simulink model "modell"  (Simulink 7.3)
settings: Solver=ode4  StartTime=0.0  StopTime=Inf  RelTol=1e-3
values from neighbouring files (symbols this model uses):
  A_w = [zeros(3) eye(3) ... (first row only)    [data.m]
  C_w = [zeros(3) eye(3)]    [data.m]
  D_i = 1*[2    0       0 ... (first row only)    [data.m]
  E_b_i = diag([1 1 1])    [data.m]
  E_b_s = diag([1 1 1])    [data.m]
  K_1 = debug*[diag([-2.2   -2.2    -2.2]) ... (first row only)    [data.m]
  K_2 = debug*0.001*diag([1 1 1])    [data.m]
  K_3 = debug*0.001*diag([0.01 0.01 0.001])    [data.m]
  K_4 = debug*0.001*diag([0.1 0.1 0.1])    [data.m]
  Ke = 100*diag([1.28 1.05 1.28 1.05 2.14])    [data.m]    (also in parameeters.m = diag([1.28 1.05 1.28 1.05 2.14]))
  M_i = 1*[25.8     0       0 ... (first row only)    [data.m]
  pos_0_i = [0, 0, 0]'    [data.m]
  pos_diff = pos_0_s - pos_0_i    [data.m]
  T_i = diag([1000, 1000, 1000])    [data.m]
  T_s = diag([1000, 1000, 1000])    [data.m]
  T_s_inv = T_s^(-1)    [data.m]
  Te = [1     0       1       0       0 ... (first row only)    [data.m]    (also in parameeters.m = [1 0 1 0 0; 0 1 0 1 1; ly1 -lx1 -ly2 -lx2 lx3])
undefined symbols (not defined in the file or in its folder): D, M
libraries: marine_gnc x13, simulink x5, simulink_extras x2
(part 1 of 2)
settings Model: Creator=mcl  LastModifiedBy=mcl  BufferReuse=off
settings OptimizationCC: BlockReduction=off  OptimizeBlockIOStorage=off  BufferReuse=off  ExpressionFolding=off  LocalBlockOutputs=off
settings RTWCC: SystemTargetFile=nidll_vxworks.tlc  TemplateMakefile=nidll_vxworks.tmf  Description=NI Real-Time VxWorks Target for Release 2007b or later  ProcessScript=nidll_vxworks_make_rtw_hook
settings STFCustomTargetCC: MatFileLogging=on  SystemTargetFile=nidll_vxworks.tlc

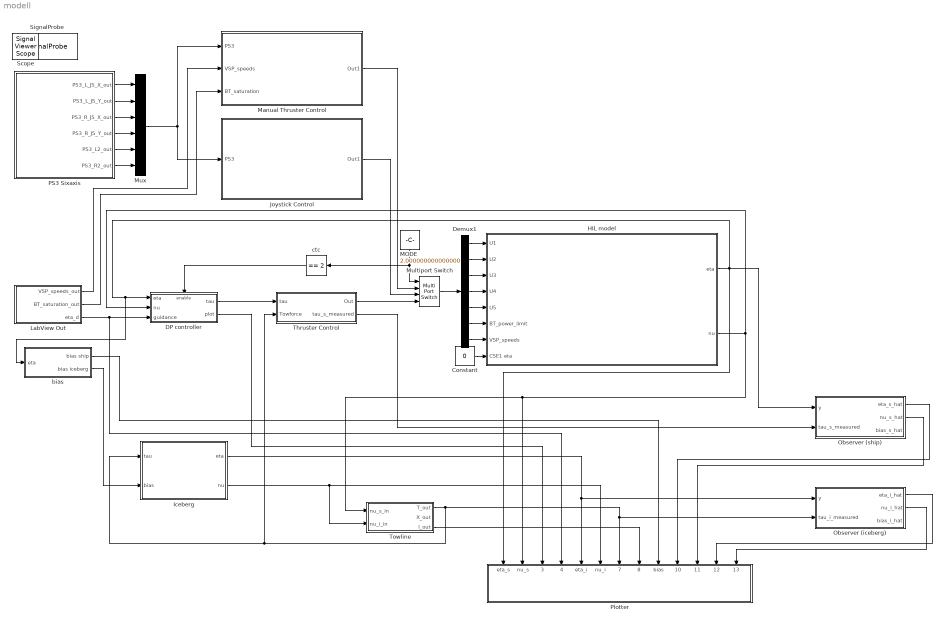
== system modell ==
  Constant : Constant  Value=0  OutDataType=fixdt(1, 16)  OutScaling=2^0
  DP controller : Subsystem
  Demux1 : Demux  Outputs=7
  HIL model : Subsystem
  Iceberg : Subsystem  AncestorBlock=marine_gnc/Examples/Vessels/CyberShipII  LoadFcn=initCS2
      mask Display:
      | image(imread('figs/cs.jpg'))
      | color('white'); port_label('output', 1, 'eta')
      | color('white');port_label('output', 2, 'nu')
      | color('white'); port_label('input', 1, 'tau')
  Joystick Control : Subsystem
  LabView Out : Subsystem
  MODE : Constant  Value=2.000000000000000  OutDataType=fixdt(1, 16)  OutScaling=2^0
  Manual Thruster Control : Subsystem
  Multiport Switch : MultiPortSwitch  zeroidx=on  OutDataType=fixdt(1, 16)  OutScaling=2^0
  Mux : Mux  Inputs=6
  Observer (iceberg) : Subsystem
  Observer (ship) : Subsystem
  PS3 Sixaxis : Subsystem
  Plotter : Subsystem
  SignalProbe : S-Function  Description=Use this block with SIT.  FunctionName=SignalProbe  Parameters=1  EnableBusSupport=off
      settings: PreSaveFcn=NISIT_ModelVars;
      mask Description: The LabVIEW Simulation Interface Toolkit uses the SignalProbe block to probe the signals in the model. The SignalProbe block must be on the top level of the model hierarchy. You can have only one SignalProbe block per model file. Do not rename the SignalProbe block. Do not change the name of another model block to SignalProbe.
  Thruster Control : Subsystem
  Towline : Subsystem
  bias : Subsystem
  ctc : simulink/Logic and Bit Operations/Compare To Constant  SystemSampleTime=-1  relop===  const=2  LogicOutDataTypeMode=uint8
  Scope : SignalViewerScope  IOType=viewer  RefreshTime=0.035000
  wires:
  Demux1/1 -> HIL model/1(U1)
  Demux1/2 -> HIL model/2(U2)
  Demux1/3 -> HIL model/3(U3)
  Demux1/4 -> HIL model/4(U4)
  Demux1/5 -> HIL model/5(U5)
  Demux1/6 -> HIL model/6(BT_power_limit)
  Demux1/7 -> HIL model/7(VSP_speeds)
  Constant/1 -> HIL model/8(CSE1 eta)
  LabView Out/3(eta_d) -> DP controller/3(guidance), Plotter/4(guidance)
  HIL model/1(eta) -> Plotter/1(eta_s), Observer (ship)/1(y), DP controller/1(eta), bias/1(eta)
  HIL model/2(nu) -> Plotter/2(nu_s), Towline/1(nu_s_in), DP controller/2(nu)
  DP controller/1(tau) -> Thruster Control/1(tau)
  DP controller/2(plot) -> Plotter/3(controller)
  Iceberg/1(eta) -> Plotter/5(eta_i), Observer (iceberg)/1(y)
  Iceberg/2(nu) -> Towline/2(nu_i_in), Plotter/6(nu_i)
  Towline/1(T_out) -> Iceberg/1(tau), Thruster Control/2(Towforce), Plotter/7(tow force), Observer (iceberg)/2(tau_i_measured)
  bias/2(bias iceberg) -> Iceberg/2(bias)
  PS3 Sixaxis/1(PS3_L_JS_X_out) -> Mux/1
  PS3 Sixaxis/2(PS3_L_JS_Y_out) -> Mux/2
  PS3 Sixaxis/3(PS3_R_JS_X_out) -> Mux/3
  PS3 Sixaxis/4(PS3_R_JS_Y_out) -> Mux/4
  PS3 Sixaxis/5(PS3_L2_out) -> Mux/5
  PS3 Sixaxis/6(PS3_R2_out) -> Mux/6
  Thruster Control/2(tau_s_measured) -> Observer (ship)/2(tau_s_measured)
  Observer (ship)/1(eta_s_hat) -> Plotter/10(eta_s_hat)
  Observer (ship)/2(nu_s_hat) -> Plotter/11(nu_s_hat)
  Multiport Switch/1 -> Demux1/1
  Thruster Control/1(Out) -> Multiport Switch/4
  MODE/1 -> Multiport Switch/1, ctc/1
  Mux/1 -> Manual Thruster Control/1(PS3), Joystick Control/1(PS3)
  LabView Out/1(VSP_speeds_out) -> Manual Thruster Control/2(VSP_speeds)
  LabView Out/2(BT_saturation_out) -> Manual Thruster Control/3(BT_saturation)
  Manual Thruster Control/1(Out1) -> Multiport Switch/2
  Joystick Control/1(Out1) -> Multiport Switch/3
  ctc/1 -> DP controller/Enable
  Towline/3(l_out) -> Plotter/8(tow length)
  bias/1(bias ship) -> Plotter/9(bias)
  Observer (iceberg)/1(eta_i_hat) -> Plotter/12(eta_i_hat)
  Observer (iceberg)/2(nu_i_hat) -> Plotter/13(nu_i_hat)

== system modell/DP controller ==
  note: eta_d
  eta : Inport  OutDataType=fixdt(1, 16)  OutScaling=2^0
  nu : Inport  Port=2  OutDataType=fixdt(1, 16)  OutScaling=2^0
  guidance : Inport  Port=3  OutDataType=fixdt(1, 16)  OutScaling=2^0
  Enable : EnablePort  StatesWhenEnabling=reset
  DP controller : Subsystem  AncestorBlock="marine_gnc/Control/Dynamic  Positioning /DP controller"  mask(Nonlinear DP Controller){Kp=(0.1)^2*[25.8000 0  0;  0  33.8000  1.0115;  0  1.0115  2.7600 ], Kd=2*0.8*0.1*[25.8000 0  0;  0  33.8000  1.0115;  0  1.0115  2.7600 ], Ki=(0.1^3/10)*[25.8000 0  0;  0  33.8000  1.0115;  0  1.0115  2.7600 ]}
      mask prompts: Kp "Proportional Gain Matrix: Kp"; Kd "Derivative Gain Matrix: Kd"; Ki "Integral Gain Matrix: Ki"
      mask help: Nonlinear PID controller for Set-Point Reulation in Surge, Sway and Yaw
      mask Help:
      | The nonlinear  PID controller uses the rotation matrix in yaw for proper scaling of the surge, sway and yaw gains as a function of the yaw angle.
      | INPUTS: (1) eta_ref, (2) eta, (3) nu. OUPUTS: (1) tau.
      mask Display: disp('Nonlinear PID\n set-point controller')
  tau : Outport  OutDataType=fixdt(1, 16)  OutScaling=2^0
  plot : Outport  Port=2  OutDataType=fixdt(1, 16)  OutScaling=2^0
  wires:
  DP controller/1(tau) -> tau/1, plot/1
  eta/1 -> DP controller/2(eta)
  nu/1 -> DP controller/3(nu)
  guidance/1 -> DP controller/1(eta_ref)

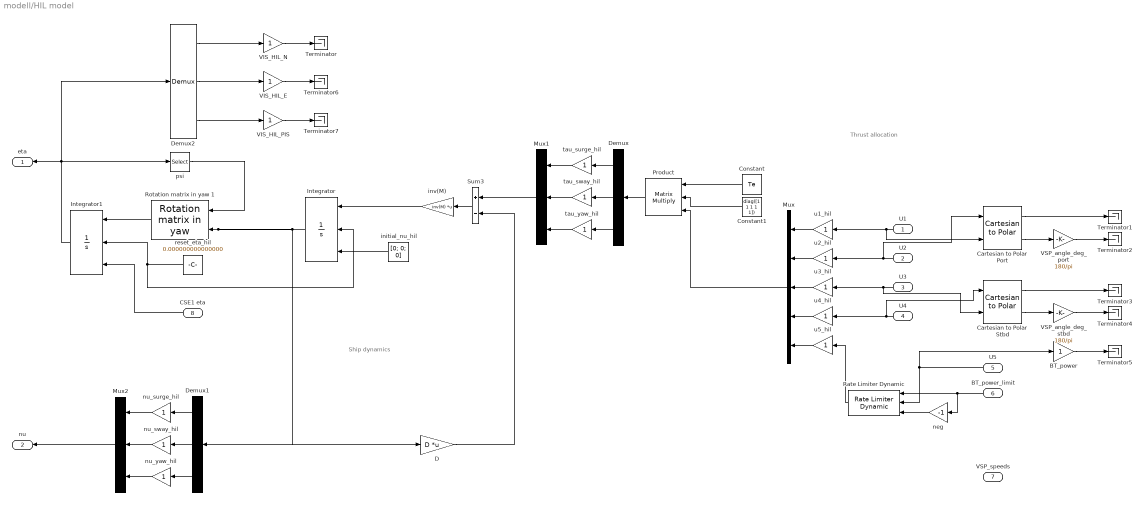
== system modell/HIL model ==
  note: Ship dynamics
  note: Thrust allocation
  U1 : Inport  OutDataType=fixdt(1, 16)  OutScaling=2^0
  U2 : Inport  Port=2  OutDataType=fixdt(1, 16)  OutScaling=2^0
  U3 : Inport  Port=3  OutDataType=fixdt(1, 16)  OutScaling=2^0
  U4 : Inport  Port=4  OutDataType=fixdt(1, 16)  OutScaling=2^0
  U5 : Inport  Port=5  OutDataType=fixdt(1, 16)  OutScaling=2^0
  BT_power_limit : Inport  Port=6  OutDataType=fixdt(1, 16)  OutScaling=2^0
  VSP_speeds : Inport  Port=7  OutDataType=fixdt(1, 16)  OutScaling=2^0
  CSE1 eta : Inport  Port=8  OutDataType=fixdt(1, 16)  OutScaling=2^0
  BT_power : Gain  ParameterDataType=fixdt(1, 16)  ParameterScaling=2^0  OutDataType=fixdt(1, 16)  OutScaling=2^0
  Cartesian to Polar Port : simulink_extras/Transformations/Cartesian to Polar  SystemSampleTime=-1
  Cartesian to Polar Stbd : simulink_extras/Transformations/Cartesian to Polar  SystemSampleTime=-1
  Constant : Constant  Value=Te
  Constant1 : Constant  Value=diag([1 1 1 1 1])
  D : Gain  Gain=D  Multiplication=Matrix(K*u)  ParameterDataType=sfix(16)  ParameterScaling=2^0  OutDataType=sfix(16)  OutScaling=2^0  SaturateOnIntegerOverflow=on  OutDataTypeStr=Inherit: Same as input  ParamDataTypeStr=Inherit: Same as input
  Demux : Demux  Outputs=3
  Demux1 : Demux  Outputs=3
  Demux2 : Demux  Outputs=3
  Integrator : Integrator  ExternalReset=level  InitialConditionSource=external
  Integrator1 : Integrator  ExternalReset=level  InitialConditionSource=external
  Mux : Mux  Inputs=5
  Mux1 : Mux  Inputs=3
  Mux2 : Mux  Inputs=3
  Product : Product  Inputs=3  Multiplication=Matrix(*)  RndMeth=Zero
  Rate Limiter Dynamic : simulink/Discontinuities/Rate Limiter Dynamic  SystemSampleTime=-1
  Rotation matrix in yaw 1 : marine_gnc/Models/ Kinematics/Rotation matrix in yaw   SystemSampleTime=-1
  Sum3 : Sum  Inputs=+-  OutDataType=sfix(16)  OutScaling=2^0  SaturateOnIntegerOverflow=on  InputSameDT=on  OutDataTypeStr=Inherit: Same as first input
  Terminator{,1..7} (8 alike) : Terminator
  VIS_HIL_E : Gain  ParameterDataType=fixdt(1, 16)  ParameterScaling=2^0  OutDataType=fixdt(1, 16)  OutScaling=2^0
  VIS_HIL_N : Gain  ParameterDataType=fixdt(1, 16)  ParameterScaling=2^0  OutDataType=fixdt(1, 16)  OutScaling=2^0
  VIS_HIL_PIS : Gain  ParameterDataType=fixdt(1, 16)  ParameterScaling=2^0  OutDataType=fixdt(1, 16)  OutScaling=2^0
  VSP_angle_deg_port : Gain  Gain=180/pi  ParameterDataType=fixdt(1, 16)  ParameterScaling=2^0  OutDataType=fixdt(1, 16)  OutScaling=2^0
  VSP_angle_deg_stbd : Gain  Gain=180/pi  ParameterDataType=fixdt(1, 16)  ParameterScaling=2^0  OutDataType=fixdt(1, 16)  OutScaling=2^0
  initial_nu_hil : Constant  Value=[0; 0; 0]  OutDataType=fixdt(1, 16)  OutScaling=2^0
  inv(M) : Gain  Gain=inv(M)  Multiplication=Matrix(K*u)  ParameterDataType=sfix(16)  ParameterScaling=2^0  OutDataType=sfix(16)  OutScaling=2^0  SaturateOnIntegerOverflow=on  OutDataTypeStr=Inherit: Same as input  ParamDataTypeStr=Inherit: Same as input
  neg : Gain  Gain=-1  ParameterDataType=fixdt(1, 16)  ParameterScaling=2^0  OutDataType=fixdt(1, 16)  OutScaling=2^0
  nu_surge_hil : Gain  ParameterDataType=fixdt(1, 16)  ParameterScaling=2^0  OutDataType=fixdt(1, 16)  OutScaling=2^0
  nu_sway_hil : Gain  ParameterDataType=fixdt(1, 16)  ParameterScaling=2^0  OutDataType=fixdt(1, 16)  OutScaling=2^0
  nu_yaw_hil : Gain  ParameterDataType=fixdt(1, 16)  ParameterScaling=2^0  OutDataType=fixdt(1, 16)  OutScaling=2^0
  psi : Selector  InputPortWidth=3  IndexOptions=Index vector (dialog)  Indices=[3]  OutputSizes=1
  reset_eta_hil : Constant  Value=0.000000000000000  OutDataType=fixdt(1, 16)  OutScaling=2^0
  tau_surge_hil : Gain  ParameterDataType=fixdt(1, 16)  ParameterScaling=2^0  OutDataType=fixdt(1, 16)  OutScaling=2^0
  tau_sway_hil : Gain  ParameterDataType=fixdt(1, 16)  ParameterScaling=2^0  OutDataType=fixdt(1, 16)  OutScaling=2^0
  tau_yaw_hil : Gain  ParameterDataType=fixdt(1, 16)  ParameterScaling=2^0  OutDataType=fixdt(1, 16)  OutScaling=2^0
  u1_hil : Gain  ParameterDataType=fixdt(1, 16)  ParameterScaling=2^0  OutDataType=fixdt(1, 16)  OutScaling=2^0
  u2_hil : Gain  ParameterDataType=fixdt(1, 16)  ParameterScaling=2^0  OutDataType=fixdt(1, 16)  OutScaling=2^0
  u3_hil : Gain  ParameterDataType=fixdt(1, 16)  ParameterScaling=2^0  OutDataType=fixdt(1, 16)  OutScaling=2^0
  u4_hil : Gain  ParameterDataType=fixdt(1, 16)  ParameterScaling=2^0  OutDataType=fixdt(1, 16)  OutScaling=2^0
  u5_hil : Gain  ParameterDataType=fixdt(1, 16)  ParameterScaling=2^0  OutDataType=fixdt(1, 16)  OutScaling=2^0
  eta : Outport  OutDataType=sfix(16)  OutScaling=2^0
  nu : Outport  Port=2  OutDataType=sfix(16)  OutScaling=2^0
  wires:
  Integrator/1 -> D/1, Demux1/1, Rotation matrix in yaw 1/2
  D/1 -> Sum3/2
  Sum3/1 -> inv(M)/1
  Rotation matrix in yaw 1/1 -> Integrator1/1
  psi/1 -> Rotation matrix in yaw 1/1
  Constant1/1 -> Product/2
  Mux/1 -> Product/3
  Constant/1 -> Product/1
  inv(M)/1 -> Integrator/1
  initial_nu_hil/1 -> Integrator/3
  U1/1 -> u1_hil/1, Cartesian to Polar Port/2
  U2/1 -> u2_hil/1, Cartesian to Polar Port/1
  U3/1 -> u3_hil/1, Cartesian to Polar Stbd/2
  U4/1 -> u4_hil/1, Cartesian to Polar Stbd/1
  Demux/1 -> tau_surge_hil/1
  tau_surge_hil/1 -> Mux1/1
  Demux/2 -> tau_sway_hil/1
  tau_sway_hil/1 -> Mux1/2
  Demux/3 -> tau_yaw_hil/1
  tau_yaw_hil/1 -> Mux1/3
  Product/1 -> Demux/1
  u1_hil/1 -> Mux/1
  u2_hil/1 -> Mux/2
  u3_hil/1 -> Mux/3
  u4_hil/1 -> Mux/4
  u5_hil/1 -> Mux/5
  Demux1/1 -> nu_surge_hil/1
  nu_surge_hil/1 -> Mux2/1
  Demux1/2 -> nu_sway_hil/1
  nu_sway_hil/1 -> Mux2/2
  Demux1/3 -> nu_yaw_hil/1
  nu_yaw_hil/1 -> Mux2/3
  Mux2/1 -> nu/1
  Mux1/1 -> Sum3/1
  Cartesian to Polar Port/1 -> Terminator1/1
  Cartesian to Polar Port/2 -> VSP_angle_deg_port/1
  VSP_angle_deg_port/1 -> Terminator2/1
  Cartesian to Polar Stbd/1 -> Terminator3/1
  Cartesian to Polar Stbd/2 -> VSP_angle_deg_stbd/1
  VSP_angle_deg_stbd/1 -> Terminator4/1
  BT_power/1 -> Terminator5/1
  Integrator1/1 -> psi/1, eta/1, Demux2/1
  reset_eta_hil/1 -> Integrator1/2, Integrator/2
  CSE1 eta/1 -> Integrator1/3
  VIS_HIL_N/1 -> Terminator/1
  Demux2/1 -> VIS_HIL_N/1
  VIS_HIL_E/1 -> Terminator6/1
  VIS_HIL_PIS/1 -> Terminator7/1
  Demux2/2 -> VIS_HIL_E/1
  Demux2/3 -> VIS_HIL_PIS/1
  Rate Limiter Dynamic/1 -> u5_hil/1
  BT_power_limit/1 -> Rate Limiter Dynamic/1, neg/1
  neg/1 -> Rate Limiter Dynamic/3
  U5/1 -> BT_power/1, Rate Limiter Dynamic/2

== system modell/Iceberg ==
  note: nu
  note: nu_dot
  note: etadot
  tau : Inport  OutDataType=sfix(16)  OutScaling=2^0
  bias : Inport  Port=2  OutDataType=fixdt(1, 16)  OutScaling=2^0
  D : Gain  Gain=D_i  Multiplication=Matrix(K*u)  ParameterDataType=sfix(16)  ParameterScaling=2^0  OutDataType=sfix(16)  OutScaling=2^0  SaturateOnIntegerOverflow=on  OutDataTypeStr=Inherit: Same as input  ParamDataTypeStr=Inherit: Same as input
  Integrator1 : Integrator  InitialConditionSource=external
  Integrator2 : Integrator
  Rotation matrix in yaw 1 : marine_gnc/Models/ Kinematics/Rotation matrix in yaw   SystemSampleTime=-1
  Sum3 : Sum  Inputs=+-+  OutDataType=sfix(16)  OutScaling=2^0  SaturateOnIntegerOverflow=on  InputSameDT=on  OutDataTypeStr=Inherit: Same as first input
  initial position : Constant  Value=pos_0_i  OutDataType=fixdt(1, 16)  OutScaling=2^0
  inv(M) : Gain  Gain=inv(M_i)  Multiplication=Matrix(K*u)  ParameterDataType=sfix(16)  ParameterScaling=2^0  OutDataType=sfix(16)  OutScaling=2^0  SaturateOnIntegerOverflow=on  OutDataTypeStr=Inherit: Same as input  ParamDataTypeStr=Inherit: Same as input
  psi : Selector  InputPortWidth=3  IndexOptions=Index vector (dialog)  Indices=[3]  OutputSizes=1
  saturation : Subsystem
  eta : Outport  OutDataType=sfix(16)  OutScaling=2^0
  nu : Outport  Port=2  OutDataType=sfix(16)  OutScaling=2^0
  wires:
  tau/1 -> saturation/1(tau)
  Integrator2/1 -> Rotation matrix in yaw 1/2, nu/1, D/1
  D/1 -> Sum3/2
  Sum3/1 -> inv(M)/1
  inv(M)/1 -> Integrator2/1
  Rotation matrix in yaw 1/1 -> Integrator1/1
  Integrator1/1 -> eta/1, psi/1
  psi/1 -> Rotation matrix in yaw 1/1
  saturation/1(sat_tau) -> Sum3/1
  initial position/1 -> Integrator1/2
  bias/1 -> Sum3/3

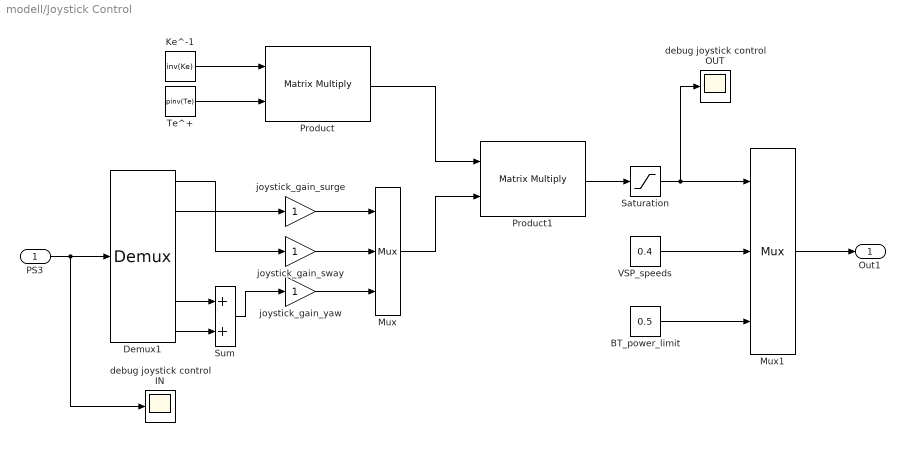
== system modell/Joystick Control ==
  PS3 : Inport  OutDataType=fixdt(1, 16)  OutScaling=2^0
  BT_power_limit : Constant  Value=0.5  OutDataType=fixdt(1, 16)  OutScaling=2^0
  Demux1 : Demux  Outputs=6
  Ke^-1 : Constant  Value=inv(Ke)  OutDataType=fixdt(1, 16)  OutScaling=2^0
  Mux : Mux  Inputs=3
  Mux1 : Mux  Inputs=3
  Product : Product  Multiplication=Matrix(*)  OutDataType=fixdt(1, 16)  OutScaling=2^0  RndMeth=Zero
  Product1 : Product  Multiplication=Matrix(*)  OutDataType=fixdt(1, 16)  OutScaling=2^0  RndMeth=Zero
  Saturation : Saturate  UpperLimit=1.0  LowerLimit=-1.0  OutDataType=fixdt(1, 16)  OutScaling=2^0
  Sum : Sum  OutDataType=fixdt(1, 16)  OutScaling=2^0
  Te^+ : Constant  Value=pinv(Te)  OutDataType=fixdt(1, 16)  OutScaling=2^0
  VSP_speeds : Constant  Value=0.4  OutDataType=fixdt(1, 16)  OutScaling=2^0
  debug joystick control IN : Scope
      settings: YMin=-1.1  YMax=1.1  SaveName=ScopeData17
  debug joystick control OUT : Scope
      settings: YMin=-0.5  YMax=0.65  SaveName=ScopeData16
  joystick_gain_surge : Gain  ParameterDataType=fixdt(1, 16)  ParameterScaling=2^0  OutDataType=fixdt(1, 16)  OutScaling=2^0
  joystick_gain_sway : Gain  ParameterDataType=fixdt(1, 16)  ParameterScaling=2^0  OutDataType=fixdt(1, 16)  OutScaling=2^0
  joystick_gain_yaw : Gain  ParameterDataType=fixdt(1, 16)  ParameterScaling=2^0  OutDataType=fixdt(1, 16)  OutScaling=2^0
  Out1 : Outport  OutDataType=fixdt(1, 16)  OutScaling=2^0
  wires:
  PS3/1 -> Demux1/1, debug joystick control IN/1
  Demux1/1 -> joystick_gain_sway/1
  Demux1/2 -> joystick_gain_surge/1
  Demux1/5 -> Sum/1
  Demux1/6 -> Sum/2
  Sum/1 -> joystick_gain_yaw/1
  Ke^-1/1 -> Product/1
  Te^+/1 -> Product/2
  Product/1 -> Product1/1
  joystick_gain_surge/1 -> Mux/1
  joystick_gain_sway/1 -> Mux/2
  joystick_gain_yaw/1 -> Mux/3
  Mux/1 -> Product1/2
  Mux1/1 -> Out1/1
  VSP_speeds/1 -> Mux1/2
  BT_power_limit/1 -> Mux1/3
  Product1/1 -> Saturation/1
  Saturation/1 -> Mux1/1, debug joystick control OUT/1

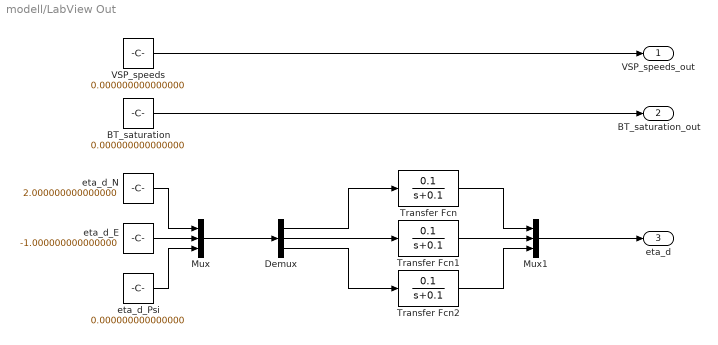
== system modell/LabView Out ==
  BT_saturation : Constant  Value=0.000000000000000  OutDataType=fixdt(1, 16)  OutScaling=2^0
  Demux : Demux  Outputs=3
  Mux : Mux  Inputs=3
  Mux1 : Mux  Inputs=3
  Transfer Fcn : TransferFcn  Numerator=[0.1]  Denominator=[1 0.1]
  Transfer Fcn1 : TransferFcn  Numerator=[0.1]  Denominator=[1 0.1]
  Transfer Fcn2 : TransferFcn  Numerator=[0.1]  Denominator=[1 0.1]
  VSP_speeds : Constant  Value=0.000000000000000  OutDataType=fixdt(1, 16)  OutScaling=2^0
  eta_d_E : Constant  Value=-1.000000000000000  OutDataType=fixdt(1, 16)  OutScaling=2^0
  eta_d_N : Constant  Value=2.000000000000000  OutDataType=fixdt(1, 16)  OutScaling=2^0
  eta_d_Psi : Constant  Value=0.000000000000000  OutDataType=fixdt(1, 16)  OutScaling=2^0
  VSP_speeds_out : Outport  OutDataType=fixdt(1, 16)  OutScaling=2^0
  BT_saturation_out : Outport  Port=2  OutDataType=fixdt(1, 16)  OutScaling=2^0
  eta_d : Outport  Port=3  OutDataType=fixdt(1, 16)  OutScaling=2^0
  wires:
  eta_d_N/1 -> Mux/1
  eta_d_E/1 -> Mux/2
  eta_d_Psi/1 -> Mux/3
  Mux/1 -> Demux/1
  Demux/3 -> Transfer Fcn2/1
  Demux/2 -> Transfer Fcn1/1
  Demux/1 -> Transfer Fcn/1
  Transfer Fcn1/1 -> Mux1/2
  Transfer Fcn2/1 -> Mux1/3
  Transfer Fcn/1 -> Mux1/1
  Mux1/1 -> eta_d/1
  VSP_speeds/1 -> VSP_speeds_out/1
  BT_saturation/1 -> BT_saturation_out/1

== system modell/Manual Thruster Control ==
  PS3 : Inport  OutDataType=fixdt(1, 16)  OutScaling=2^0
  VSP_speeds : Inport  Port=2  OutDataType=fixdt(1, 16)  OutScaling=2^0
  BT_saturation : Inport  Port=3  OutDataType=fixdt(1, 16)  OutScaling=2^0
  Demux1 : Demux  Outputs=6
  Mux : Mux  Inputs=7
  Sum : Sum  OutDataType=fixdt(1, 16)  OutScaling=2^0
  U{1..5} (5 alike) : Gain  ParameterDataType=fixdt(1, 16)  ParameterScaling=2^0  OutDataType=fixdt(1, 16)  OutScaling=2^0
  Out1 : Outport  OutDataType=fixdt(1, 16)  OutScaling=2^0
  wires:
  Mux/1 -> Out1/1
  PS3/1 -> Demux1/1
  Demux1/5 -> Sum/1
  Demux1/6 -> Sum/2
  Sum/1 -> U5/1
  BT_saturation/1 -> Mux/6
  VSP_speeds/1 -> Mux/7
  U1/1 -> Mux/1
  U2/1 -> Mux/2
  U3/1 -> Mux/3
  U4/1 -> Mux/4
  U5/1 -> Mux/5
  Demux1/2 -> U1/1
  Demux1/1 -> U2/1
  Demux1/4 -> U3/1
  Demux1/3 -> U4/1

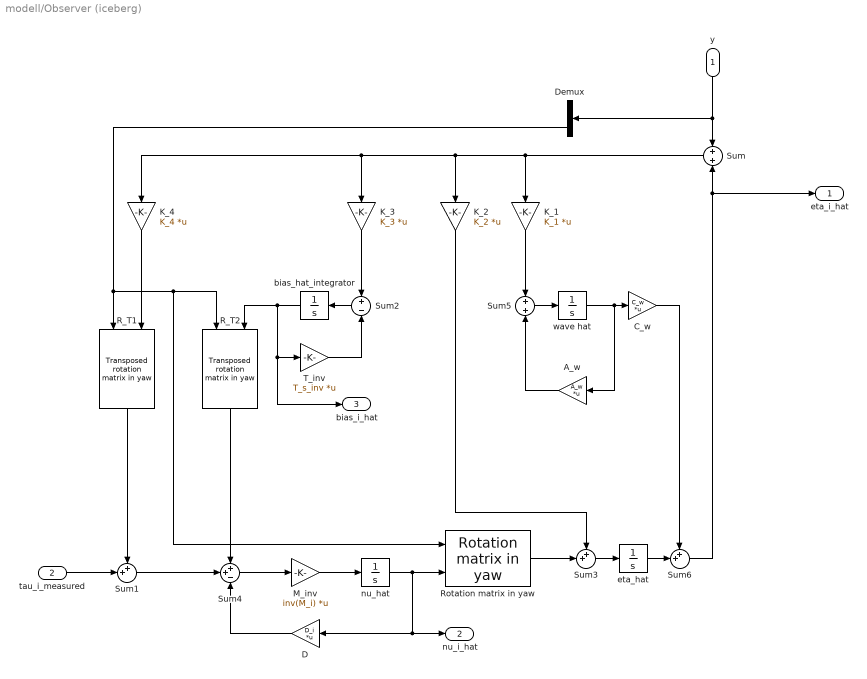
== system modell/Observer (iceberg) ==
  y : Inport  OutDataType=fixdt(1, 16)  OutScaling=2^0
  tau_i_measured : Inport  Port=2  OutDataType=fixdt(1, 16)  OutScaling=2^0
  A_w : Gain  Gain=A_w  Multiplication=Matrix(K*u)  ParameterDataType=fixdt(1, 16)  ParameterScaling=2^0  OutDataType=fixdt(1, 16)  OutScaling=2^0
  C_w : Gain  Gain=C_w  Multiplication=Matrix(K*u)  ParameterDataType=fixdt(1, 16)  ParameterScaling=2^0  OutDataType=fixdt(1, 16)  OutScaling=2^0
  D : Gain  Gain=D_i  Multiplication=Matrix(K*u)  ParameterDataType=fixdt(1, 16)  ParameterScaling=2^0  OutDataType=fixdt(1, 16)  OutScaling=2^0
  Demux : Demux  Outputs=3
  K_1 : Gain  Gain=K_1  Multiplication=Matrix(K*u)  ParameterDataType=fixdt(1, 16)  ParameterScaling=2^0  OutDataType=fixdt(1, 16)  OutScaling=2^0
  K_2 : Gain  Gain=K_2  Multiplication=Matrix(K*u)  ParameterDataType=fixdt(1, 16)  ParameterScaling=2^0  OutDataType=fixdt(1, 16)  OutScaling=2^0
  K_3 : Gain  Gain=K_3  Multiplication=Matrix(K*u)  ParameterDataType=fixdt(1, 16)  ParameterScaling=2^0  OutDataType=fixdt(1, 16)  OutScaling=2^0
  K_4 : Gain  Gain=K_4  Multiplication=Matrix(K*u)  ParameterDataType=fixdt(1, 16)  ParameterScaling=2^0  OutDataType=fixdt(1, 16)  OutScaling=2^0
  M_inv : Gain  Gain=inv(M_i)  Multiplication=Matrix(K*u)  ParameterDataType=fixdt(1, 16)  ParameterScaling=2^0  OutDataType=fixdt(1, 16)  OutScaling=2^0
  R_T1 : marine_gnc/Models/ Kinematics/Transposed rotation  matrix in yaw  SystemSampleTime=-1
  R_T2 : marine_gnc/Models/ Kinematics/Transposed rotation  matrix in yaw  SystemSampleTime=-1
  "Rotation matrix in yaw " : marine_gnc/Models/ Kinematics/Rotation matrix in yaw   SystemSampleTime=-1
  Sum : Sum  OutDataType=fixdt(1, 16)  OutScaling=2^0
  Sum1 : Sum  Inputs=++|  OutDataType=fixdt(1, 16)  OutScaling=2^0
  Sum2 : Sum  Inputs=+-  OutDataType=fixdt(1, 16)  OutScaling=2^0
  Sum3 : Sum  Inputs=++|  OutDataType=fixdt(1, 16)  OutScaling=2^0
  Sum4 : Sum  Inputs=++-  OutDataType=fixdt(1, 16)  OutScaling=2^0
  Sum5 : Sum  OutDataType=fixdt(1, 16)  OutScaling=2^0
  Sum6 : Sum  Inputs=++|  OutDataType=fixdt(1, 16)  OutScaling=2^0
  T_inv : Gain  Gain=T_s_inv  Multiplication=Matrix(K*u)  ParameterDataType=fixdt(1, 16)  ParameterScaling=2^0  OutDataType=fixdt(1, 16)  OutScaling=2^0
  bias_hat_integrator : Integrator
  eta_hat : Integrator
  nu_hat : Integrator
  wave hat : Integrator
  eta_i_hat : Outport  OutDataType=fixdt(1, 16)  OutScaling=2^0
  nu_i_hat : Outport  Port=2  OutDataType=fixdt(1, 16)  OutScaling=2^0
  bias_i_hat : Outport  Port=3  OutDataType=fixdt(1, 16)  OutScaling=2^0
  wires:
  tau_i_measured/1 -> Sum1/2
  y/1 -> Sum/1, Demux/1
  Sum/1 -> K_4/1, K_3/1, K_2/1, K_1/1
  K_4/1 -> R_T1/2
  R_T1/1 -> Sum1/1
  Demux/3 -> R_T1/1, R_T2/1, "Rotation matrix in yaw "/1
  R_T2/1 -> Sum4/1
  Sum1/1 -> Sum4/2
  K_3/1 -> Sum2/1
  T_inv/1 -> Sum2/2
  Sum2/1 -> bias_hat_integrator/1
  bias_hat_integrator/1 -> R_T2/2, T_inv/1, bias_i_hat/1
  Sum4/1 -> M_inv/1
  M_inv/1 -> nu_hat/1
  nu_hat/1 -> "Rotation matrix in yaw "/2, D/1, nu_i_hat/1
  D/1 -> Sum4/3
  "Rotation matrix in yaw "/1 -> Sum3/2
  K_2/1 -> Sum3/1
  K_1/1 -> Sum5/1
  Sum5/1 -> wave hat/1
  A_w/1 -> Sum5/2
  wave hat/1 -> C_w/1, A_w/1
  Sum3/1 -> eta_hat/1
  eta_hat/1 -> Sum6/2
  Sum6/1 -> Sum/2, eta_i_hat/1
  C_w/1 -> Sum6/1

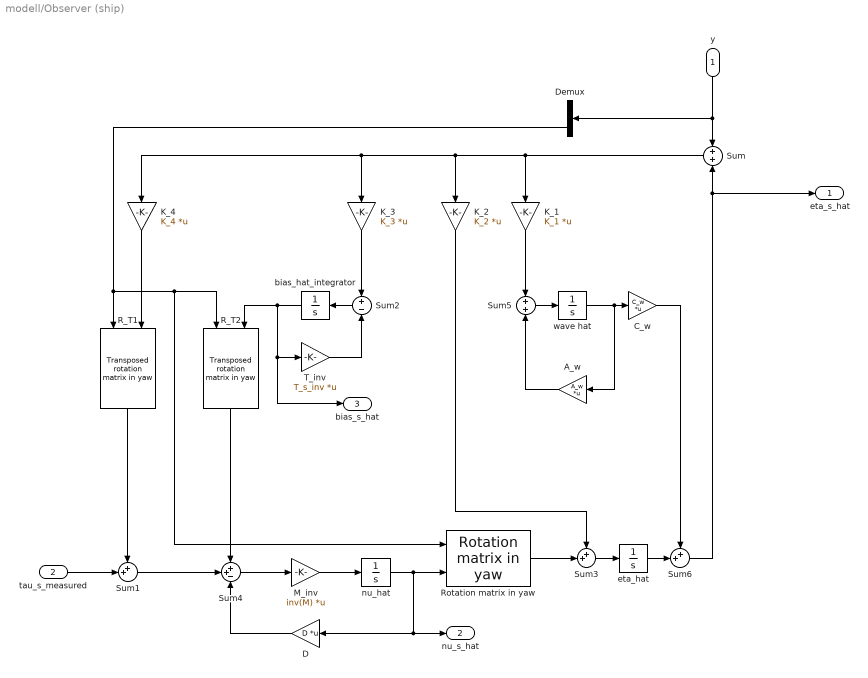
== system modell/Observer (ship) ==
  y : Inport  OutDataType=fixdt(1, 16)  OutScaling=2^0
  tau_s_measured : Inport  Port=2  OutDataType=fixdt(1, 16)  OutScaling=2^0
  A_w : Gain  Gain=A_w  Multiplication=Matrix(K*u)  ParameterDataType=fixdt(1, 16)  ParameterScaling=2^0  OutDataType=fixdt(1, 16)  OutScaling=2^0
  C_w : Gain  Gain=C_w  Multiplication=Matrix(K*u)  ParameterDataType=fixdt(1, 16)  ParameterScaling=2^0  OutDataType=fixdt(1, 16)  OutScaling=2^0
  D : Gain  Gain=D  Multiplication=Matrix(K*u)  ParameterDataType=fixdt(1, 16)  ParameterScaling=2^0  OutDataType=fixdt(1, 16)  OutScaling=2^0
  Demux : Demux  Outputs=3
  K_1 : Gain  Gain=K_1  Multiplication=Matrix(K*u)  ParameterDataType=fixdt(1, 16)  ParameterScaling=2^0  OutDataType=fixdt(1, 16)  OutScaling=2^0
  K_2 : Gain  Gain=K_2  Multiplication=Matrix(K*u)  ParameterDataType=fixdt(1, 16)  ParameterScaling=2^0  OutDataType=fixdt(1, 16)  OutScaling=2^0
  K_3 : Gain  Gain=K_3  Multiplication=Matrix(K*u)  ParameterDataType=fixdt(1, 16)  ParameterScaling=2^0  OutDataType=fixdt(1, 16)  OutScaling=2^0
  K_4 : Gain  Gain=K_4  Multiplication=Matrix(K*u)  ParameterDataType=fixdt(1, 16)  ParameterScaling=2^0  OutDataType=fixdt(1, 16)  OutScaling=2^0
  M_inv : Gain  Gain=inv(M)  Multiplication=Matrix(K*u)  ParameterDataType=fixdt(1, 16)  ParameterScaling=2^0  OutDataType=fixdt(1, 16)  OutScaling=2^0
  R_T1 : marine_gnc/Models/ Kinematics/Transposed rotation  matrix in yaw  SystemSampleTime=-1
  R_T2 : marine_gnc/Models/ Kinematics/Transposed rotation  matrix in yaw  SystemSampleTime=-1
  "Rotation matrix in yaw " : marine_gnc/Models/ Kinematics/Rotation matrix in yaw   SystemSampleTime=-1
  Sum : Sum  OutDataType=fixdt(1, 16)  OutScaling=2^0
  Sum1 : Sum  Inputs=++|  OutDataType=fixdt(1, 16)  OutScaling=2^0
  Sum2 : Sum  Inputs=+-  OutDataType=fixdt(1, 16)  OutScaling=2^0
  Sum3 : Sum  Inputs=++|  OutDataType=fixdt(1, 16)  OutScaling=2^0
  Sum4 : Sum  Inputs=++-  OutDataType=fixdt(1, 16)  OutScaling=2^0
  Sum5 : Sum  OutDataType=fixdt(1, 16)  OutScaling=2^0
  Sum6 : Sum  Inputs=++|  OutDataType=fixdt(1, 16)  OutScaling=2^0
  T_inv : Gain  Gain=T_s_inv  Multiplication=Matrix(K*u)  ParameterDataType=fixdt(1, 16)  ParameterScaling=2^0  OutDataType=fixdt(1, 16)  OutScaling=2^0
  bias_hat_integrator : Integrator
  eta_hat : Integrator
  nu_hat : Integrator
  wave hat : Integrator
  eta_s_hat : Outport  OutDataType=fixdt(1, 16)  OutScaling=2^0
  nu_s_hat : Outport  Port=2  OutDataType=fixdt(1, 16)  OutScaling=2^0
  bias_s_hat : Outport  Port=3  OutDataType=fixdt(1, 16)  OutScaling=2^0
  wires:
  tau_s_measured/1 -> Sum1/2
  y/1 -> Sum/1, Demux/1
  Sum/1 -> K_4/1, K_3/1, K_2/1, K_1/1
  K_4/1 -> R_T1/2
  R_T1/1 -> Sum1/1
  Demux/3 -> R_T1/1, R_T2/1, "Rotation matrix in yaw "/1
  R_T2/1 -> Sum4/1
  Sum1/1 -> Sum4/2
  K_3/1 -> Sum2/1
  T_inv/1 -> Sum2/2
  Sum2/1 -> bias_hat_integrator/1
  bias_hat_integrator/1 -> R_T2/2, T_inv/1, bias_s_hat/1
  Sum4/1 -> M_inv/1
  M_inv/1 -> nu_hat/1
  nu_hat/1 -> "Rotation matrix in yaw "/2, D/1, nu_s_hat/1
  D/1 -> Sum4/3
  "Rotation matrix in yaw "/1 -> Sum3/2
  K_2/1 -> Sum3/1
  K_1/1 -> Sum5/1
  Sum5/1 -> wave hat/1
  A_w/1 -> Sum5/2
  wave hat/1 -> C_w/1, A_w/1
  Sum3/1 -> eta_hat/1
  eta_hat/1 -> Sum6/2
  Sum6/1 -> Sum/2, eta_s_hat/1
  C_w/1 -> Sum6/1

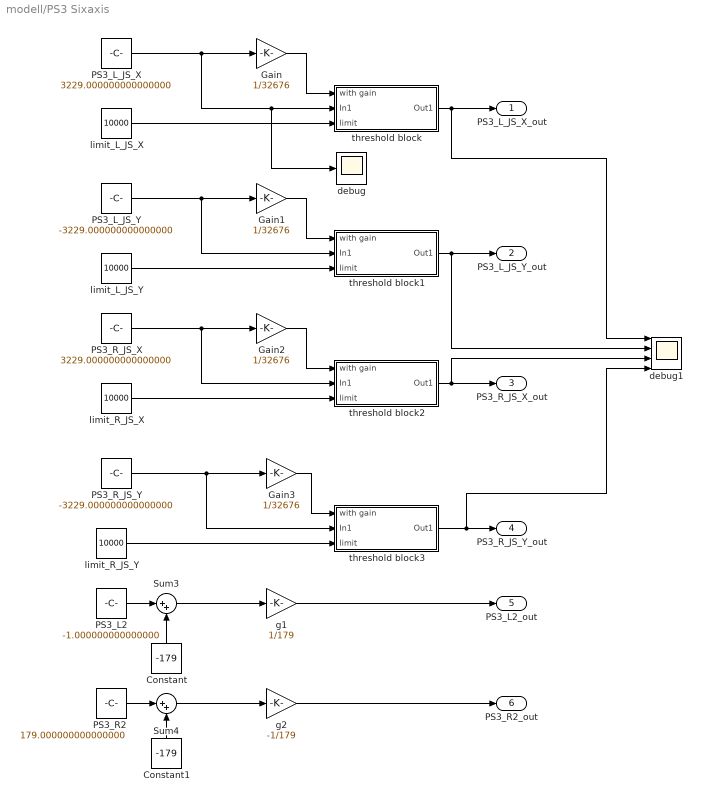
== system modell/PS3 Sixaxis ==
  Constant : Constant  Value=-179  OutDataType=fixdt(1, 16)  OutScaling=2^0
  Constant1 : Constant  Value=-179  OutDataType=fixdt(1, 16)  OutScaling=2^0
  Gain{,1..3} (4 alike) : Gain  Gain=1/32676  ParameterDataType=fixdt(1, 16)  ParameterScaling=2^0  OutDataType=fixdt(1, 16)  OutScaling=2^0
  PS3_L2 : Constant  Value=-1.000000000000000  OutDataType=fixdt(1, 16)  OutScaling=2^0
  PS3_L_JS_X : Constant  Value=3229.000000000000000  OutDataType=fixdt(1, 16)  OutScaling=2^0
  PS3_L_JS_Y : Constant  Value=-3229.000000000000000  OutDataType=fixdt(1, 16)  OutScaling=2^0
  PS3_R2 : Constant  Value=179.000000000000000  OutDataType=fixdt(1, 16)  OutScaling=2^0
  PS3_R_JS_X : Constant  Value=3229.000000000000000  OutDataType=fixdt(1, 16)  OutScaling=2^0
  PS3_R_JS_Y : Constant  Value=-3229.000000000000000  OutDataType=fixdt(1, 16)  OutScaling=2^0
  Sum3 : Sum  Inputs=|++  OutDataType=fixdt(1, 16)  OutScaling=2^0
  Sum4 : Sum  Inputs=|++  OutDataType=fixdt(1, 16)  OutScaling=2^0
  debug : Scope
      settings: YMin=3513  YMax=3513  SaveName=ScopeData9
  debug1 : Scope  NumInputPorts=4
      settings: YMin=-1~-1~-1~-1  YMax=1~1~1~1  SaveName=ScopeData10
  g1 : Gain  Gain=1/179  ParameterDataType=fixdt(1, 16)  ParameterScaling=2^0  OutDataType=fixdt(1, 16)  OutScaling=2^0
  g2 : Gain  Gain=-1/179  ParameterDataType=fixdt(1, 16)  ParameterScaling=2^0  OutDataType=fixdt(1, 16)  OutScaling=2^0
  limit_L_JS_X : Constant  Value=10000  OutDataType=fixdt(1, 16)  OutScaling=2^0
  limit_L_JS_Y : Constant  Value=10000  OutDataType=fixdt(1, 16)  OutScaling=2^0
  limit_R_JS_X : Constant  Value=10000  OutDataType=fixdt(1, 16)  OutScaling=2^0
  limit_R_JS_Y : Constant  Value=10000  OutDataType=fixdt(1, 16)  OutScaling=2^0
  threshold block : Subsystem
  threshold block1 : Subsystem
  threshold block2 : Subsystem
  threshold block3 : Subsystem
  PS3_L_JS_X_out : Outport  OutDataType=fixdt(1, 16)  OutScaling=2^0
  PS3_L_JS_Y_out : Outport  Port=2  OutDataType=fixdt(1, 16)  OutScaling=2^0
  PS3_R_JS_X_out : Outport  Port=3  OutDataType=fixdt(1, 16)  OutScaling=2^0
  PS3_R_JS_Y_out : Outport  Port=4  OutDataType=fixdt(1, 16)  OutScaling=2^0
  PS3_L2_out : Outport  Port=5  OutDataType=fixdt(1, 16)  OutScaling=2^0
  PS3_R2_out : Outport  Port=6  OutDataType=fixdt(1, 16)  OutScaling=2^0
  wires:
  PS3_L_JS_Y/1 -> Gain1/1, threshold block1/2(In1)
  PS3_L_JS_X/1 -> Gain/1, threshold block/2(In1), debug/1
  PS3_R_JS_Y/1 -> Gain3/1, threshold block3/2(In1)
  PS3_R_JS_X/1 -> Gain2/1, threshold block2/2(In1)
  PS3_L2/1 -> Sum3/1
  Sum3/1 -> g1/1
  PS3_R2/1 -> Sum4/1
  Sum4/1 -> g2/1
  threshold block/1(Out1) -> debug1/1, PS3_L_JS_X_out/1
  Gain/1 -> threshold block/1(with gain)
  Gain1/1 -> threshold block1/1(with gain)
  threshold block1/1(Out1) -> debug1/2, PS3_L_JS_Y_out/1
  Gain2/1 -> threshold block2/1(with gain)
  threshold block2/1(Out1) -> debug1/3, PS3_R_JS_X_out/1
  Gain3/1 -> threshold block3/1(with gain)
  threshold block3/1(Out1) -> debug1/4, PS3_R_JS_Y_out/1
  limit_L_JS_X/1 -> threshold block/3(limit)
  limit_L_JS_Y/1 -> threshold block1/3(limit)
  limit_R_JS_X/1 -> threshold block2/3(limit)
  limit_R_JS_Y/1 -> threshold block3/3(limit)
  g1/1 -> PS3_L2_out/1
  g2/1 -> PS3_R2_out/1
  Constant/1 -> Sum3/2
  Constant1/1 -> Sum4/2

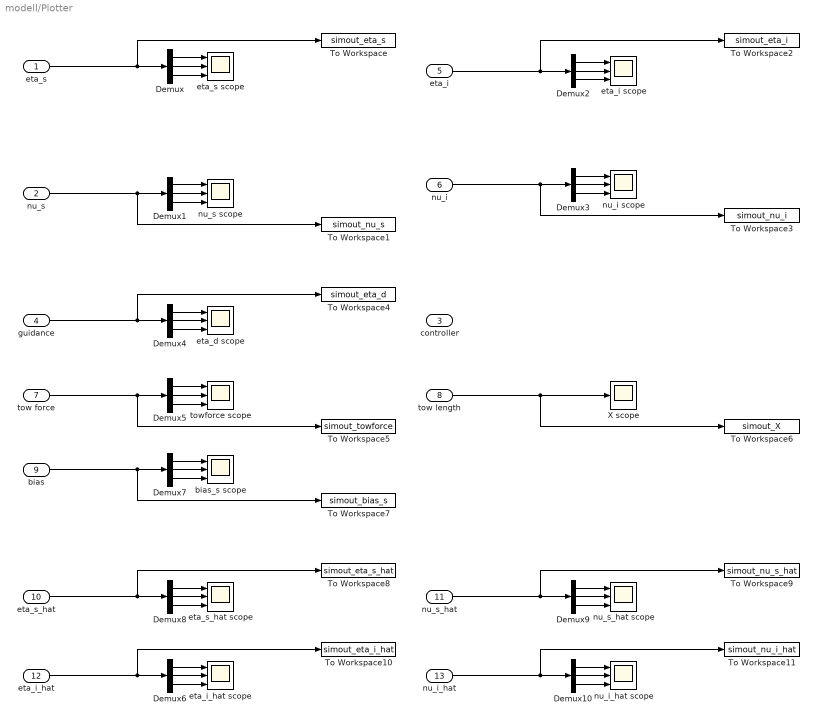
== system modell/Plotter ==
  eta_s : Inport  OutDataType=fixdt(1, 16)  OutScaling=2^0
  nu_s : Inport  Port=2  OutDataType=fixdt(1, 16)  OutScaling=2^0
  controller : Inport  Port=3  OutDataType=fixdt(1, 16)  OutScaling=2^0
  guidance : Inport  Port=4  OutDataType=fixdt(1, 16)  OutScaling=2^0
  eta_i : Inport  Port=5  OutDataType=fixdt(1, 16)  OutScaling=2^0
  nu_i : Inport  Port=6  OutDataType=fixdt(1, 16)  OutScaling=2^0
  tow force : Inport  Port=7  OutDataType=fixdt(1, 16)  OutScaling=2^0
  tow length : Inport  Port=8  OutDataType=fixdt(1, 16)  OutScaling=2^0
  bias : Inport  Port=9  OutDataType=fixdt(1, 16)  OutScaling=2^0
  eta_s_hat : Inport  Port=10  OutDataType=fixdt(1, 16)  OutScaling=2^0
  nu_s_hat : Inport  Port=11  OutDataType=fixdt(1, 16)  OutScaling=2^0
  eta_i_hat : Inport  Port=12  OutDataType=fixdt(1, 16)  OutScaling=2^0
  nu_i_hat : Inport  Port=13  OutDataType=fixdt(1, 16)  OutScaling=2^0
  Demux{,1..10} (11 alike) : Demux  Outputs=3
  To Workspace : ToWorkspace  VariableName=simout_eta_s  SampleTime=-1  SaveFormat=Structure With Time
  To Workspace1 : ToWorkspace  VariableName=simout_nu_s  SampleTime=-1  SaveFormat=Structure
  To Workspace10 : ToWorkspace  VariableName=simout_eta_i_hat  SampleTime=-1  SaveFormat=Structure
  To Workspace11 : ToWorkspace  VariableName=simout_nu_i_hat  SampleTime=-1  SaveFormat=Structure
  To Workspace2 : ToWorkspace  VariableName=simout_eta_i  SampleTime=-1  SaveFormat=Structure
  To Workspace3 : ToWorkspace  VariableName=simout_nu_i  SampleTime=-1  SaveFormat=Structure
  To Workspace4 : ToWorkspace  VariableName=simout_eta_d  SampleTime=-1  SaveFormat=Structure
  To Workspace5 : ToWorkspace  VariableName=simout_towforce  SampleTime=-1  SaveFormat=Structure
  To Workspace6 : ToWorkspace  VariableName=simout_X  SampleTime=-1  SaveFormat=Structure
  To Workspace7 : ToWorkspace  VariableName=simout_bias_s  SampleTime=-1  SaveFormat=Structure
  To Workspace8 : ToWorkspace  VariableName=simout_eta_s_hat  SampleTime=-1  SaveFormat=Structure
  To Workspace9 : ToWorkspace  VariableName=simout_nu_s_hat  SampleTime=-1  SaveFormat=Structure
  X scope : Scope
      settings: YMin=10  YMax=30  SaveName=ScopeData6
  bias_s scope : Scope  NumInputPorts=3
      settings: YMin=-2.5~-2.5~-2.5  YMax=0.75~0.75~0.75  SaveName=ScopeData8
  eta_d scope : Scope  NumInputPorts=3
      settings: YMin=-5~-5~-5  YMax=5~5~5  SaveName=ScopeData4
  eta_i scope : Scope  NumInputPorts=3
      settings: YMin=-5~-5~-5  YMax=5~5~5  SaveName=ScopeData2
  eta_i_hat scope : Scope  NumInputPorts=3
      settings: YMin=8.55~-0.0015~-0.00225  YMax=9.45~0.001~0.0025  SaveName=ScopeData14
  eta_s scope : Scope  NumInputPorts=3
      settings: YMin=8.55~-0.0015~-0.00225  YMax=9.45~0.001~0.0025
  eta_s_hat scope : Scope  NumInputPorts=3
      settings: YMin=8.55~-0.0015~-0.00225  YMax=9.45~0.001~0.0025  SaveName=ScopeData11
  nu_i scope : Scope  NumInputPorts=3
      settings: YMin=-5~-5~-5  YMax=5~5~5  SaveName=ScopeData3
  nu_i_hat scope : Scope  NumInputPorts=3
      settings: YMin=8.55~-0.0015~-0.00225  YMax=9.45~0.001~0.0025  SaveName=ScopeData15
  nu_s scope : Scope  NumInputPorts=3
      settings: YMin=-5~-5~-5  YMax=5~5~5
  nu_s_hat scope : Scope  NumInputPorts=3
      settings: YMin=8.55~-0.0015~-0.00225  YMax=9.45~0.001~0.0025  SaveName=ScopeData12
  towforce scope : Scope  NumInputPorts=3
      settings: YMin=9~-3.51e-021~-1  YMax=27~-3.47e-021~1  SaveName=ScopeData5
  wires:
  eta_s/1 -> Demux/1, To Workspace/1
  Demux/1 -> eta_s scope/1
  Demux/2 -> eta_s scope/2
  Demux/3 -> eta_s scope/3
  nu_s/1 -> Demux1/1, To Workspace1/1
  Demux1/1 -> nu_s scope/1
  Demux1/2 -> nu_s scope/2
  Demux1/3 -> nu_s scope/3
  eta_i/1 -> Demux2/1, To Workspace2/1
  Demux2/1 -> eta_i scope/1
  Demux2/2 -> eta_i scope/2
  Demux2/3 -> eta_i scope/3
  nu_i/1 -> Demux3/1, To Workspace3/1
  Demux3/1 -> nu_i scope/1
  Demux3/2 -> nu_i scope/2
  Demux3/3 -> nu_i scope/3
  guidance/1 -> Demux4/1, To Workspace4/1
  Demux4/1 -> eta_d scope/1
  Demux4/2 -> eta_d scope/2
  Demux4/3 -> eta_d scope/3
  tow force/1 -> Demux5/1, To Workspace5/1
  Demux5/1 -> towforce scope/1
  Demux5/2 -> towforce scope/2
  Demux5/3 -> towforce scope/3
  tow length/1 -> To Workspace6/1, X scope/1
  bias/1 -> Demux7/1, To Workspace7/1
  Demux7/1 -> bias_s scope/1
  Demux7/2 -> bias_s scope/2
  Demux7/3 -> bias_s scope/3
  eta_s_hat/1 -> Demux8/1, To Workspace8/1
  Demux8/1 -> eta_s_hat scope/1
  Demux8/2 -> eta_s_hat scope/2
  Demux8/3 -> eta_s_hat scope/3
  nu_s_hat/1 -> Demux9/1, To Workspace9/1
  Demux9/1 -> nu_s_hat scope/1
  Demux9/2 -> nu_s_hat scope/2
  Demux9/3 -> nu_s_hat scope/3
  eta_i_hat/1 -> Demux6/1, To Workspace10/1
  Demux6/1 -> eta_i_hat scope/1
  Demux6/2 -> eta_i_hat scope/2
  Demux6/3 -> eta_i_hat scope/3
  nu_i_hat/1 -> Demux10/1, To Workspace11/1
  Demux10/1 -> nu_i_hat scope/1
  Demux10/2 -> nu_i_hat scope/2
  Demux10/3 -> nu_i_hat scope/3

== system modell/Thruster Control ==
  tau : Inport  OutDataType=fixdt(1, 16)  OutScaling=2^0
  Towforce : Inport  Port=2  OutDataType=fixdt(1, 16)  OutScaling=2^0
  BT_power_limit : Constant  Value=0.5  OutDataType=fixdt(1, 16)  OutScaling=2^0
  Ke^-1 : Constant  Value=inv(Ke)  OutDataType=fixdt(1, 16)  OutScaling=2^0
  Mux1 : Mux  Inputs=3
  Product : Product  Multiplication=Matrix(*)  OutDataType=fixdt(1, 16)  OutScaling=2^0  RndMeth=Zero
  Product1 : Product  Multiplication=Matrix(*)  OutDataType=fixdt(1, 16)  OutScaling=2^0  RndMeth=Zero
  Saturation : Saturate  UpperLimit=1.0  LowerLimit=-1.0  OutDataType=fixdt(1, 16)  OutScaling=2^0
  Sum : Sum  Inputs=|+-  OutDataType=fixdt(1, 16)  OutScaling=2^0
  Te^+ : Constant  Value=pinv(Te)  OutDataType=fixdt(1, 16)  OutScaling=2^0
  VSP_speeds : Constant  Value=0.4  OutDataType=fixdt(1, 16)  OutScaling=2^0
  Out : Outport  OutDataType=fixdt(1, 16)  OutScaling=2^0
  tau_s_measured : Outport  Port=2  OutDataType=fixdt(1, 16)  OutScaling=2^0
  wires:
  Mux1/1 -> Out/1
  Ke^-1/1 -> Product/1
  Te^+/1 -> Product/2
  Product1/1 -> Saturation/1
  VSP_speeds/1 -> Mux1/2
  BT_power_limit/1 -> Mux1/3
  Saturation/1 -> Mux1/1
  Product/1 -> Product1/1
  tau/1 -> Sum/1
  Sum/1 -> Product1/2, tau_s_measured/1
  Towforce/1 -> Sum/2

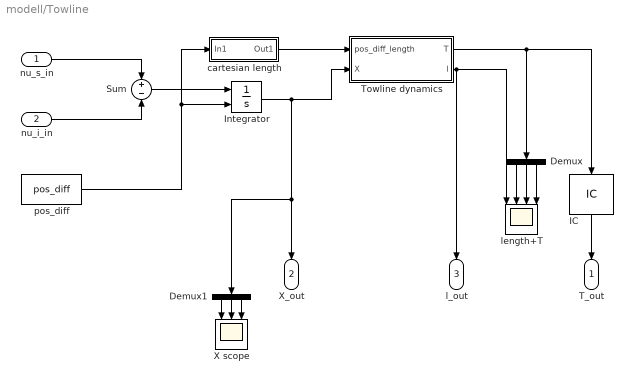
== system modell/Towline ==
  nu_s_in : Inport  OutDataType=fixdt(1, 16)  OutScaling=2^0
  nu_i_in : Inport  Port=2  OutDataType=fixdt(1, 16)  OutScaling=2^0
  Demux : Demux  Outputs=3
  Demux1 : Demux  Outputs=3
  IC : InitialCondition  Value=[0 0 0]'
  Integrator : Integrator  InitialConditionSource=external
  Sum : Sum  Inputs=+-  OutDataType=fixdt(1, 16)  OutScaling=2^0
  Towline dynamics : Subsystem
  X scope : Scope  NumInputPorts=3
      settings: YMin=0~0~0  YMax=350~35000~7500  SaveName=ScopeData13
  cartesian length : Subsystem
  length+T : Scope  NumInputPorts=4
      settings: YMin=0~0~0~-0.55  YMax=350~35000~7500~0.2  SaveName=ScopeData7
  pos_diff : Constant  Value=pos_diff  OutDataType=fixdt(1, 16)  OutScaling=2^0
  T_out : Outport  OutDataType=fixdt(1, 16)  OutScaling=2^0
  X_out : Outport  Port=2  OutDataType=fixdt(1, 16)  OutScaling=2^0
  l_out : Outport  Port=3  OutDataType=fixdt(1, 16)  OutScaling=2^0
  wires:
  nu_s_in/1 -> Sum/1
  nu_i_in/1 -> Sum/2
  Sum/1 -> Integrator/1
  pos_diff/1 -> Integrator/2, cartesian length/1(In1)
  Integrator/1 -> Towline dynamics/2(X), X_out/1, Demux1/1
  Towline dynamics/1(T) -> IC/1, Demux/1
  IC/1 -> T_out/1
  Demux/3 -> length+T/4
  Demux/2 -> length+T/3
  Demux/1 -> length+T/2
  Towline dynamics/2(l) -> length+T/1, l_out/1
  cartesian length/1(Out1) -> Towline dynamics/1(pos_diff_length)
  Demux1/3 -> X scope/3
  Demux1/2 -> X scope/2
  Demux1/1 -> X scope/1

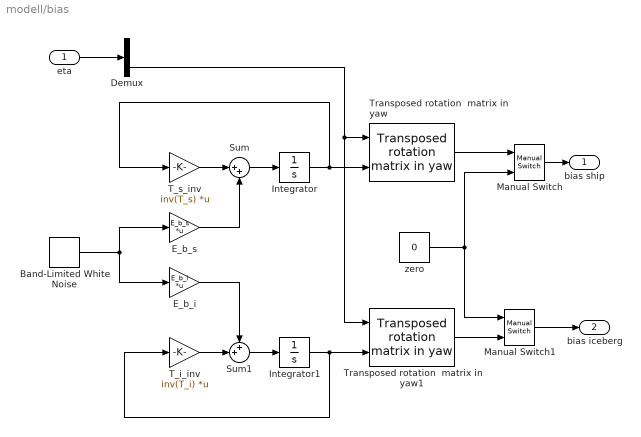
== system modell/bias ==
  eta : Inport  OutDataType=fixdt(1, 16)  OutScaling=2^0
  Band-Limited White Noise : simulink/Sources/Band-Limited White Noise  SystemSampleTime=-1  Cov=[0.01 0.01 0.001]  Ts=0.1  seed=[23341]
  Demux : Demux  Outputs=3
  E_b_i : Gain  Gain=E_b_i  Multiplication=Matrix(K*u)  ParameterDataType=fixdt(1, 16)  ParameterScaling=2^0  OutDataType=fixdt(1, 16)  OutScaling=2^0
  E_b_s : Gain  Gain=E_b_s  Multiplication=Matrix(K*u)  ParameterDataType=fixdt(1, 16)  ParameterScaling=2^0  OutDataType=fixdt(1, 16)  OutScaling=2^0
  Integrator : Integrator
  Integrator1 : Integrator
  Manual Switch : simulink/Signal Routing/Manual Switch  SystemSampleTime=-1  sw=0  action=0  varsize=off
  Manual Switch1 : simulink/Signal Routing/Manual Switch  SystemSampleTime=-1  sw=1  action=0  varsize=off
  Sum : Sum  Inputs=|++  OutDataType=fixdt(1, 16)  OutScaling=2^0
  Sum1 : Sum  Inputs=++|  OutDataType=fixdt(1, 16)  OutScaling=2^0
  T_i_inv : Gain  Gain=inv(T_i)  Multiplication=Matrix(K*u)  ParameterDataType=fixdt(1, 16)  ParameterScaling=2^0  OutDataType=fixdt(1, 16)  OutScaling=2^0
  T_s_inv : Gain  Gain=inv(T_s)  Multiplication=Matrix(K*u)  ParameterDataType=fixdt(1, 16)  ParameterScaling=2^0  OutDataType=fixdt(1, 16)  OutScaling=2^0
  Transposed rotation  matrix in yaw : marine_gnc/Models/ Kinematics/Transposed rotation  matrix in yaw  SystemSampleTime=-1
  Transposed rotation  matrix in yaw1 : marine_gnc/Models/ Kinematics/Transposed rotation  matrix in yaw  SystemSampleTime=-1
  zero : Constant  Value=0  OutDataType=fixdt(1, 16)  OutScaling=2^0
  bias ship : Outport  OutDataType=fixdt(1, 16)  OutScaling=2^0
  bias iceberg : Outport  Port=2  OutDataType=fixdt(1, 16)  OutScaling=2^0
  wires:
  Integrator1/1 -> T_i_inv/1, Transposed rotation  matrix in yaw1/2
  Integrator/1 -> T_s_inv/1, Transposed rotation  matrix in yaw/2
  T_s_inv/1 -> Sum/1
  Sum/1 -> Integrator/1
  Band-Limited White Noise/1 -> E_b_s/1, E_b_i/1
  E_b_s/1 -> Sum/2
  Sum1/1 -> Integrator1/1
  T_i_inv/1 -> Sum1/2
  E_b_i/1 -> Sum1/1
  eta/1 -> Demux/1
  Demux/3 -> Transposed rotation  matrix in yaw/1, Transposed rotation  matrix in yaw1/1
  Manual Switch1/1 -> bias iceberg/1
  Manual Switch/1 -> bias ship/1
  Transposed rotation  matrix in yaw/1 -> Manual Switch/1
  Transposed rotation  matrix in yaw1/1 -> Manual Switch1/2
  zero/1 -> Manual Switch/2, Manual Switch1/1

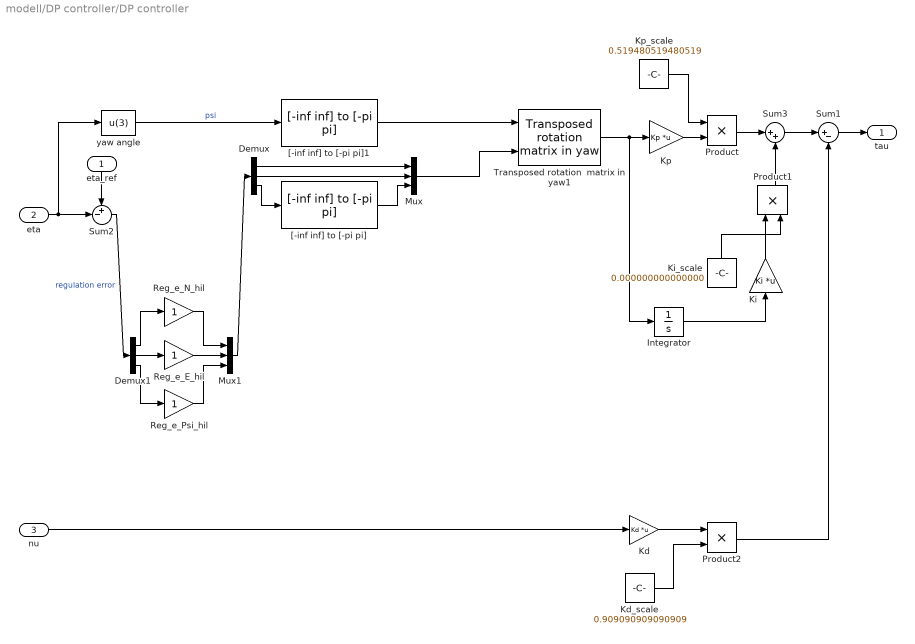
== system modell/DP controller/DP controller ==
  eta_ref : Inport  OutDataType=sfix(16)  OutScaling=2^0
  eta : Inport  Port=2  OutDataType=sfix(16)  OutScaling=2^0
  nu : Inport  Port=3  OutDataType=sfix(16)  OutScaling=2^0
  Demux : Demux  Outputs=3
  Demux1 : Demux  Outputs=3
  Integrator : Integrator
  Kd : Gain  Gain=Kd  Multiplication=Matrix(K*u)  ParameterDataType=sfix(16)  ParameterScaling=2^0  OutDataType=sfix(16)  OutScaling=2^0  SaturateOnIntegerOverflow=on  OutDataTypeStr=Inherit: Same as input  ParamDataTypeStr=Inherit: Same as input
  Kd_scale : Constant  Value=0.909090909090909  OutDataType=fixdt(1, 16)  OutScaling=2^0
  Ki : Gain  Gain=Ki  Multiplication=Matrix(K*u)  ParameterDataType=sfix(16)  ParameterScaling=2^0  OutDataType=sfix(16)  OutScaling=2^0  SaturateOnIntegerOverflow=on  OutDataTypeStr=Inherit: Same as input  ParamDataTypeStr=Inherit: Same as input
  Ki_scale : Constant  Value=0.000000000000000  OutDataType=fixdt(1, 16)  OutScaling=2^0
  Kp : Gain  Gain=Kp  Multiplication=Matrix(K*u)  ParameterDataType=sfix(16)  ParameterScaling=2^0  OutDataType=sfix(16)  OutScaling=2^0  SaturateOnIntegerOverflow=on  OutDataTypeStr=Inherit: Same as input  ParamDataTypeStr=Inherit: Same as input
  Kp_scale : Constant  Value=0.519480519480519  OutDataType=fixdt(1, 16)  OutScaling=2^0
  Mux : Mux  Inputs=3
  Mux1 : Mux  Inputs=3
  Product : Product  OutDataType=fixdt(1, 16)  OutScaling=2^0  RndMeth=Zero
  Product1 : Product  OutDataType=fixdt(1, 16)  OutScaling=2^0  RndMeth=Zero
  Product2 : Product  OutDataType=fixdt(1, 16)  OutScaling=2^0  RndMeth=Zero
  Reg_e_E_hil : Gain  ParameterDataType=fixdt(1, 16)  ParameterScaling=2^0  OutDataType=fixdt(1, 16)  OutScaling=2^0
  Reg_e_N_hil : Gain  ParameterDataType=fixdt(1, 16)  ParameterScaling=2^0  OutDataType=fixdt(1, 16)  OutScaling=2^0
  Reg_e_Psi_hil : Gain  ParameterDataType=fixdt(1, 16)  ParameterScaling=2^0  OutDataType=fixdt(1, 16)  OutScaling=2^0
  Sum1 : Sum  Inputs=|+-  OutDataType=sfix(16)  OutScaling=2^0  SaturateOnIntegerOverflow=on  InputSameDT=on  OutDataTypeStr=Inherit: Same as first input
  Sum2 : Sum  Inputs=+-|  OutDataType=sfix(16)  OutScaling=2^0  SaturateOnIntegerOverflow=on  InputSameDT=on  OutDataTypeStr=Inherit: Same as first input
  Sum3 : Sum  Inputs=|++  OutDataType=sfix(16)  OutScaling=2^0  SaturateOnIntegerOverflow=on  InputSameDT=on  OutDataTypeStr=Inherit: Same as first input
  Transposed rotation  matrix in yaw1 : marine_gnc/Models/ Kinematics/Transposed rotation  matrix in yaw  SystemSampleTime=-1
  "[-inf inf] to [-pi pi]" : marine_gnc/Utilities/Math Operations/[-inf inf] to [-pi pi]  SystemSampleTime=-1
  "[-inf inf] to [-pi pi]1" : marine_gnc/Utilities/Math Operations/[-inf inf] to [-pi pi]  SystemSampleTime=-1
  yaw angle : Fcn  Expr=u(3)
  tau : Outport  OutDataType=sfix(16)  OutScaling=2^0  InitialOutput=0
  wires:
  "[-inf inf] to [-pi pi]1"/1 -> Transposed rotation  matrix in yaw1/1
  yaw angle/1 -> "[-inf inf] to [-pi pi]1"/1  "psi"
  Mux/1 -> Transposed rotation  matrix in yaw1/2
  Demux/1 -> Mux/1
  Demux/2 -> Mux/2
  "[-inf inf] to [-pi pi]"/1 -> Mux/3
  Demux/3 -> "[-inf inf] to [-pi pi]"/1
  eta_ref/1 -> Sum2/1
  Sum1/1 -> tau/1
  eta/1 -> Sum2/2, yaw angle/1
  nu/1 -> Kd/1
  Integrator/1 -> Ki/1
  Sum3/1 -> Sum1/1
  Transposed rotation  matrix in yaw1/1 -> Kp/1, Integrator/1
  Sum2/1 -> Demux1/1  "regulation error"
  Mux1/1 -> Demux/1
  Demux1/2 -> Reg_e_E_hil/1
  Reg_e_E_hil/1 -> Mux1/2
  Demux1/1 -> Reg_e_N_hil/1
  Reg_e_N_hil/1 -> Mux1/1
  Reg_e_Psi_hil/1 -> Mux1/3
  Demux1/3 -> Reg_e_Psi_hil/1
  Kp/1 -> Product/2
  Product/1 -> Sum3/1
  Kp_scale/1 -> Product/1
  Ki/1 -> Product1/1
  Ki_scale/1 -> Product1/2
  Product1/1 -> Sum3/2
  Product2/1 -> Sum1/2
  Kd/1 -> Product2/1
  Kd_scale/1 -> Product2/2

== system modell/Iceberg/saturation ==
  tau : Inport  OutDataType=sfix(16)  OutScaling=2^0
  Demux : Demux  Outputs=3
  Mux1 : Mux  Inputs=3
  Saturation : Saturate  UpperLimit=2  LowerLimit=-2
  Saturation1 : Saturate  UpperLimit=1.5  LowerLimit=-1.5
  Saturation2 : Saturate  UpperLimit=1.5  LowerLimit=-1.5
  sat_tau : Outport  OutDataType=sfix(16)  OutScaling=2^0
  wires:
  Saturation2/1 -> Mux1/3
  Saturation1/1 -> Mux1/2
  Saturation/1 -> Mux1/1
  Demux/3 -> Saturation2/1
  Demux/2 -> Saturation1/1
  Demux/1 -> Saturation/1
  tau/1 -> Demux/1
  Mux1/1 -> sat_tau/1

== system modell/PS3 Sixaxis/threshold block ==
  with gain : Inport  OutDataType=fixdt(1, 16)  OutScaling=2^0
  In1 : Inport  Port=2  OutDataType=fixdt(1, 16)  OutScaling=2^0
  limit : Inport  Port=3  OutDataType=fixdt(1, 16)  OutScaling=2^0
  Abs : Abs  OutDataType=fixdt(1, 16)  OutScaling=2^0
  Constant2 : Constant  Value=0  OutDataType=fixdt(1, 16)  OutScaling=2^0
  If : If  NumInputs=2  IfExpression=u1 < u2
  Sum : Sum  OutDataType=fixdt(1, 16)  OutScaling=2^0
  else : Subsystem  TreatAsAtomicUnit=on
  if : Subsystem  TreatAsAtomicUnit=on
  Out1 : Outport  OutDataType=fixdt(1, 16)  OutScaling=2^0
  wires:
  If/1 -> if/Action
  Constant2/1 -> if/1(In1)
  If/2 -> else/Action
  In1/1 -> Abs/1
  Sum/1 -> Out1/1
  with gain/1 -> else/1(In1)
  if/1(Out1) -> Sum/1
  else/1(Out1) -> Sum/2
  limit/1 -> If/2
  Abs/1 -> If/1

== system modell/PS3 Sixaxis/threshold block1 ==
  with gain : Inport  OutDataType=fixdt(1, 16)  OutScaling=2^0
  In1 : Inport  Port=2  OutDataType=fixdt(1, 16)  OutScaling=2^0
  limit : Inport  Port=3  OutDataType=fixdt(1, 16)  OutScaling=2^0
  Abs : Abs  OutDataType=fixdt(1, 16)  OutScaling=2^0
  Constant2 : Constant  Value=0  OutDataType=fixdt(1, 16)  OutScaling=2^0
  If : If  NumInputs=2  IfExpression=u1 < u2
  Sum : Sum  OutDataType=fixdt(1, 16)  OutScaling=2^0
  else : Subsystem  TreatAsAtomicUnit=on
  if : Subsystem  TreatAsAtomicUnit=on
  Out1 : Outport  OutDataType=fixdt(1, 16)  OutScaling=2^0
  wires:
  If/1 -> if/Action
  Constant2/1 -> if/1(In1)
  If/2 -> else/Action
  In1/1 -> Abs/1
  Sum/1 -> Out1/1
  with gain/1 -> else/1(In1)
  if/1(Out1) -> Sum/1
  else/1(Out1) -> Sum/2
  limit/1 -> If/2
  Abs/1 -> If/1

== system modell/PS3 Sixaxis/threshold block2 ==
  with gain : Inport  OutDataType=fixdt(1, 16)  OutScaling=2^0
  In1 : Inport  Port=2  OutDataType=fixdt(1, 16)  OutScaling=2^0
  limit : Inport  Port=3  OutDataType=fixdt(1, 16)  OutScaling=2^0
  Abs : Abs  OutDataType=fixdt(1, 16)  OutScaling=2^0
  Constant2 : Constant  Value=0  OutDataType=fixdt(1, 16)  OutScaling=2^0
  If : If  NumInputs=2  IfExpression=u1 < u2
  Sum : Sum  OutDataType=fixdt(1, 16)  OutScaling=2^0
  else : Subsystem  TreatAsAtomicUnit=on
  if : Subsystem  TreatAsAtomicUnit=on
  Out1 : Outport  OutDataType=fixdt(1, 16)  OutScaling=2^0
  wires:
  If/1 -> if/Action
  Constant2/1 -> if/1(In1)
  If/2 -> else/Action
  In1/1 -> Abs/1
  Sum/1 -> Out1/1
  with gain/1 -> else/1(In1)
  if/1(Out1) -> Sum/1
  else/1(Out1) -> Sum/2
  limit/1 -> If/2
  Abs/1 -> If/1

== system modell/PS3 Sixaxis/threshold block3 ==
  with gain : Inport  OutDataType=fixdt(1, 16)  OutScaling=2^0
  In1 : Inport  Port=2  OutDataType=fixdt(1, 16)  OutScaling=2^0
  limit : Inport  Port=3  OutDataType=fixdt(1, 16)  OutScaling=2^0
  Abs : Abs  OutDataType=fixdt(1, 16)  OutScaling=2^0
  Constant2 : Constant  Value=0  OutDataType=fixdt(1, 16)  OutScaling=2^0
  If : If  NumInputs=2  IfExpression=u1 < u2
  Sum : Sum  OutDataType=fixdt(1, 16)  OutScaling=2^0
  else : Subsystem  TreatAsAtomicUnit=on
  if : Subsystem  TreatAsAtomicUnit=on
  Out1 : Outport  OutDataType=fixdt(1, 16)  OutScaling=2^0
  wires:
  If/1 -> if/Action
  Constant2/1 -> if/1(In1)
  If/2 -> else/Action
  In1/1 -> Abs/1
  Sum/1 -> Out1/1
  with gain/1 -> else/1(In1)
  if/1(Out1) -> Sum/1
  else/1(Out1) -> Sum/2
  limit/1 -> If/2
  Abs/1 -> If/1

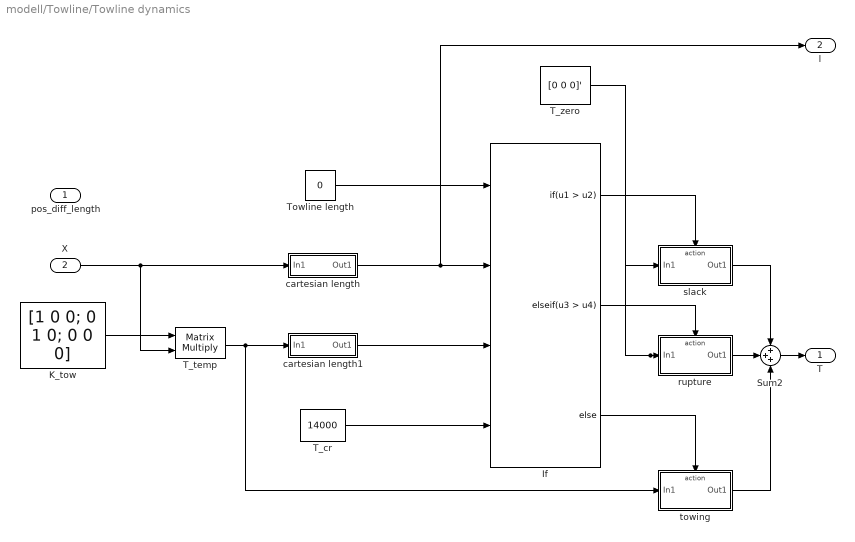
== system modell/Towline/Towline dynamics ==
  pos_diff_length : Inport  OutDataType=fixdt(1, 16)  OutScaling=2^0
  X : Inport  Port=2  OutDataType=fixdt(1, 16)  OutScaling=2^0
  If : If  NumInputs=4  IfExpression=u1 > u2  ElseIfExpressions=u3 > u4
  K_tow : Constant  Value=[1 0 0; 0 1 0; 0 0 0]  OutDataType=fixdt(1, 16)  OutScaling=2^0
  Sum2 : Sum  Inputs=+++  OutDataType=fixdt(1, 16)  OutScaling=2^0
  T_cr : Constant  Value=14000  OutDataType=fixdt(1, 16)  OutScaling=2^0
  T_temp : Product  Multiplication=Matrix(*)  OutDataType=fixdt(1, 16)  OutScaling=2^0  RndMeth=Zero
  T_zero : Constant  Value=[0 0 0]'  OutDataType=fixdt(1, 16)  OutScaling=2^0
  Towline length : Constant  Value=0  OutDataType=fixdt(1, 16)  OutScaling=2^0
  cartesian length : Subsystem
  cartesian length1 : Subsystem
  rupture : Subsystem  TreatAsAtomicUnit=on
  slack : Subsystem  TreatAsAtomicUnit=on
  towing : Subsystem  TreatAsAtomicUnit=on
  T : Outport  OutDataType=fixdt(1, 16)  OutScaling=2^0
  l : Outport  Port=2  OutDataType=fixdt(1, 16)  OutScaling=2^0
  wires:
  X/1 -> T_temp/2, cartesian length/1(In1)
  cartesian length/1(Out1) -> If/2, l/1
  Towline length/1 -> If/1
  T_temp/1 -> towing/1(In1), cartesian length1/1(In1)
  cartesian length1/1(Out1) -> If/3
  T_cr/1 -> If/4
  If/1 -> slack/Action
  If/2 -> rupture/Action
  If/3 -> towing/Action
  T_zero/1 -> slack/1(In1), rupture/1(In1)
  Sum2/1 -> T/1
  slack/1(Out1) -> Sum2/1
  rupture/1(Out1) -> Sum2/2
  towing/1(Out1) -> Sum2/3
  K_tow/1 -> T_temp/1

== system modell/Towline/cartesian length ==
  In1 : Inport  OutDataType=fixdt(1, 16)  OutScaling=2^0
  Demux : Demux  Outputs=3
  Sum : Sum  OutDataType=fixdt(1, 16)  OutScaling=2^0
  mf1 : Math  Operator=square  OutDataType=fixdt(1, 16)  OutScaling=2^0  SaturateOnIntegerOverflow=on
  mf2 : Math  Operator=square  OutDataType=fixdt(1, 16)  OutScaling=2^0  SaturateOnIntegerOverflow=on
  mf3 : Math  Operator=sqrt  OutDataType=fixdt(1, 16)  OutScaling=2^0  SaturateOnIntegerOverflow=on
  Out1 : Outport  OutDataType=fixdt(1, 16)  OutScaling=2^0
  wires:
  In1/1 -> Demux/1
  Demux/1 -> mf1/1
  Demux/2 -> mf2/1
  mf2/1 -> Sum/2
  mf1/1 -> Sum/1
  Sum/1 -> mf3/1
  mf3/1 -> Out1/1

== system modell/PS3 Sixaxis/threshold block/else ==
  In1 : Inport  OutDataType=fixdt(1, 16)  OutScaling=2^0
  Action Port : ActionPort  ActionType=else
  Out1 : Outport  OutDataType=fixdt(1, 16)  OutScaling=2^0
  wires:
  In1/1 -> Out1/1

== system modell/PS3 Sixaxis/threshold block/if ==
  In1 : Inport  OutDataType=fixdt(1, 16)  OutScaling=2^0
  Action Port : ActionPort  ActionType=then
  Out1 : Outport  OutDataType=fixdt(1, 16)  OutScaling=2^0
  wires:
  In1/1 -> Out1/1

== system modell/PS3 Sixaxis/threshold block1/else ==
  In1 : Inport  OutDataType=fixdt(1, 16)  OutScaling=2^0
  Action Port : ActionPort  ActionType=else
  Out1 : Outport  OutDataType=fixdt(1, 16)  OutScaling=2^0
  wires:
  In1/1 -> Out1/1

== system modell/PS3 Sixaxis/threshold block1/if ==
  In1 : Inport  OutDataType=fixdt(1, 16)  OutScaling=2^0
  Action Port : ActionPort  ActionType=then
  Out1 : Outport  OutDataType=fixdt(1, 16)  OutScaling=2^0
  wires:
  In1/1 -> Out1/1
